simulink model "Apps_Model"  (R2019a)
settings: Solver=VariableStepAuto  StartTime=0.0  StopTime=10.0  RelTol=1e-3
PreLoadFcn:
  | AppsInit
StopFcn:
  | AppsVisualize
settings Model: Creator=G5  LastModifiedBy=G5
settings DataIOCC: LoadExternalInput=on  SaveFormat=Array  InspectSignalLogs=on

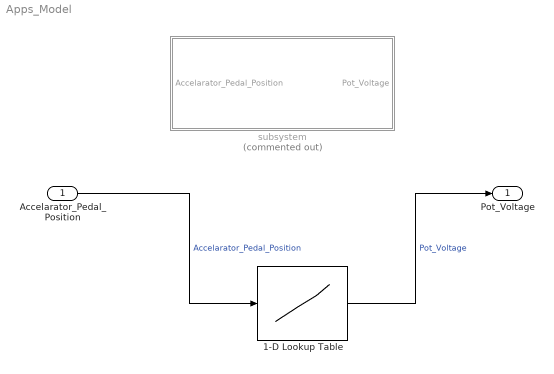
== system Apps_Model ==
  Accelarator_Pedal_Position : Inport
  1-D Lookup Table : Lookup_n-D  NumberOfTableDimensions=1  BreakpointsForDimension1=[0,0.1,0.2,0.3,0.4,0.5,0.6,0.7,0.8,0.9,1]  Table=[0.5,0.9,1.3,1.7,2.1,2.5,2.9,3.3,3.7,4.1,4.5]  InternalRulePriority=Speed  RndMeth=Simplest  InputSameDT=on
  subsystem : Subsystem  Commented=on
      mask help: App
      settings: CloseFcn=AppsVisualize
  Pot_Voltage : Outport
  wires:
  Accelarator_Pedal_Position/1 -> 1-D Lookup Table/1  "Accelarator_Pedal_Position"
  1-D Lookup Table/1 -> Pot_Voltage/1  "Pot_Voltage"

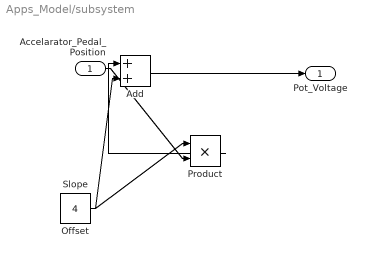
== system Apps_Model/subsystem ==
  Accelarator_Pedal_Position : Inport
  Add : Sum
  Offset : Constant  Value=0.5
  Product : Product
  Slope : Constant  Value=4
  Pot_Voltage : Outport
  wires:
  Slope/1 -> Product/1
  Accelarator_Pedal_Position/1 -> Product/2
  Product/1 -> Add/1
  Offset/1 -> Add/2
  Add/1 -> Pot_Voltage/1
